simulink model "robust_model_closed_loop"  (R2023b)
settings: Solver=VariableStepAuto  StartTime=0.0  StopTime=20  MaxStep=0.01  RelTol=1e-5
undefined symbols (not defined in the file): B_alt, E_alt, Je_inv
libraries: cstblocks x6
settings Model: Creator=torb  LastModifiedBy=torb
settings OptimizationCC: DefaultParameterBehavior=Inlined  BufferReuse=off
settings DebuggingCC: InitInArrayFormatMsg=none

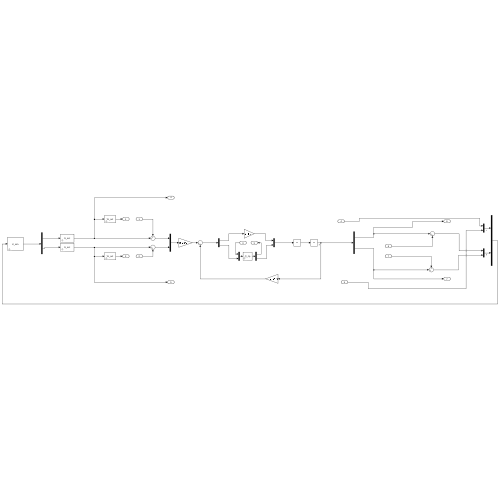
[thumbnail: Simulink's stored preview of the top-level diagram]
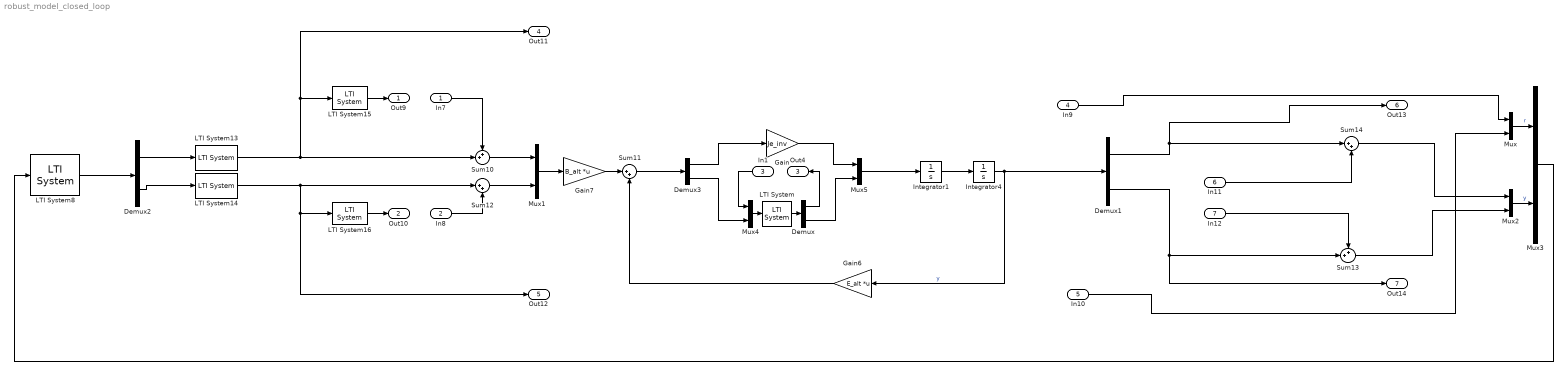
== system robust_model_closed_loop ==
  In7 : Inport
  In8 : Inport  Port=2
  In1 : Inport  Port=3
  In9 : Inport  Port=4
  In10 : Inport  Port=5
  In11 : Inport  Port=6
  In12 : Inport  Port=7
  Demux{,1..3} (4 alike) : Demux  Outputs=2
  Gain : Gain  Gain=Je_inv
  Gain6 : Gain  Gain=E_alt  Multiplication=Matrix(K*u)
  Gain7 : Gain  Gain=B_alt  Multiplication=Matrix(K*u)
  Integrator1 : Integrator
  Integrator4 : Integrator
  LTI System : cstblocks/LTI System  sys=Q_Jp  IC=[]  PadeOrder=0
  LTI System13 : cstblocks/LTI System  sys=G_act  IC=[]  PadeOrder=0
  LTI System14 : cstblocks/LTI System  sys=G_act  IC=[]  PadeOrder=0
  LTI System15 : cstblocks/LTI System  sys=W_act  IC=[]  PadeOrder=0
  LTI System16 : cstblocks/LTI System  sys=W_act  IC=[]  PadeOrder=0
  LTI System8 : cstblocks/LTI System  sys=K_sim  IC=[]  PadeOrder=0
  Mux{,1..5} (6 alike) : Mux  Inputs=2
  Sum10 : Sum  Inputs=++|
  Sum11 : Sum  Inputs=|++
  Sum12 : Sum  Inputs=|++
  Sum13 : Sum  Inputs=++|
  Sum14 : Sum  Inputs=|++
  Out9 : Outport
  Out10 : Outport  Port=2
  Out4 : Outport  Port=3
  Out11 : Outport  Port=4
  Out12 : Outport  Port=5
  Out13 : Outport  Port=6
  Out14 : Outport  Port=7
  wires:
  Demux1/1 -> Sum14/1, Out13/1
  Gain6/1 -> Sum11/2
  Sum10/1 -> Mux1/1
  In8/1 -> Sum12/2
  Integrator4/1 -> Demux1/1, Gain6/1  "y"
  Mux3/1 -> LTI System8/1
  In12/1 -> Sum13/1
  Mux1/1 -> Gain7/1
  Demux2/1 -> LTI System13/1
  Demux2/2 -> LTI System14/1
  In11/1 -> Sum14/2
  In7/1 -> Sum10/1
  LTI System16/1 -> Out10/1
  LTI System14/1 -> Sum12/1, Out12/1, LTI System16/1
  In9/1 -> Mux/1
  LTI System8/1 -> Demux2/1
  Gain7/1 -> Sum11/1
  Sum12/1 -> Mux1/2
  In10/1 -> Mux/2
  LTI System13/1 -> Sum10/2, Out11/1, LTI System15/1
  LTI System15/1 -> Out9/1
  Integrator1/1 -> Integrator4/1
  Demux1/2 -> Out14/1, Sum13/2
  Mux2/1 -> Mux3/2  "y"
  Sum13/1 -> Mux2/2
  Sum14/1 -> Mux2/1
  Mux/1 -> Mux3/1  "r"
  LTI System/1 -> Demux/1
  Mux5/1 -> Integrator1/1
  Sum11/1 -> Demux3/1
  Demux/1 -> Out4/1
  Demux3/2 -> Mux4/2
  Demux/2 -> Mux5/2
  Demux3/1 -> Gain/1
  In1/1 -> Mux4/1
  Gain/1 -> Mux5/1
  Mux4/1 -> LTI System/1
